simulink model "PMSMSim"  (R2024b)
settings: Solver=FixedStepAuto  StartTime=0  StopTime=15000  RelTol=1e-3
model workspace (MAT data in the model file):
  time = -1
libraries: deeplib x1
settings Model: SimulationMode=accelerator  Creator=skeshavm  LastModifiedBy=msatra
settings SolverCC: AlgebraicLoopSolver=TrustRegion
settings DataIOCC: SaveFormat=StructureWithTime  SaveOutput=off  SignalLogging=off  DSMLogging=off  SaveTime=off
settings OptimizationCC: DefaultParameterBehavior=Inlined  UseDivisionForNetSlopeComputation=on  GainParamInheritBuiltInType=on  UseFloatMulNetSlope=on  InlineInvariantSignals=on  StrengthReduction=on  PassReuseOutputArgsThreshold=0  ZeroExternalMemoryAtStartup=off  ZeroInternalMemoryAtStartup=off  InitFltsAndDblsToZero=on  EfficientFloat2IntCast=on  OptimizeBlockOrder=speed  OptimizationPriority=Speed  OptimizationCustomize=off  MultiThreadedLoops=on  AutoScheduleForLoops=on  DenormalBehavior=FlushToZero
settings DebuggingCC: InheritedTsInSrcMsg=none  MultiTaskCondExecSysMsg=none  MultiTaskRateTransMsg=warning  ParameterTunabilityLossMsg=error  UnconnectedInputMsg=warning  UnconnectedOutputMsg=warning  UnconnectedLineMsg=warning
settings HardwareCC: ProdLongLongMode=on  TargetLongLongMode=on
settings ModelReferenceCC: EnableRefExpFcnMdlSchedulingChecks=on
settings SFSimCC: MATLABDynamicMemAlloc=off  SimTargetLang=C++  GPUAcceleration=on  SimDLTargetLibrary=cudnn
settings RTWCC: Toolchain=Microsoft Visual C++ 2019 v16.0 | nmake (64-bit Windows)  BuildConfiguration=Faster Runs  TargetLang=C++  CheckMdlBeforeBuild=Warning  GPUErrorChecks=on  GPUComputeCapability=7.5  DLArmComputeVersion=19.05
settings CodeAppCC: ForceParamTrailComments=on  OperatorAnnotations=on
settings GRTTargetCC: TargetLangStandard=C++11 (ISO)  CodeInterfacePackaging=C++ class

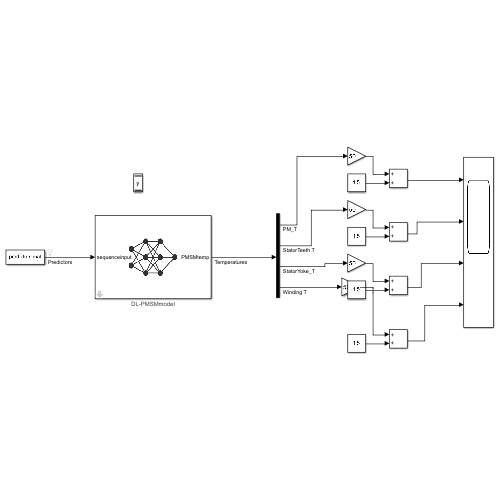
[thumbnail: Simulink's stored preview of the top-level diagram]
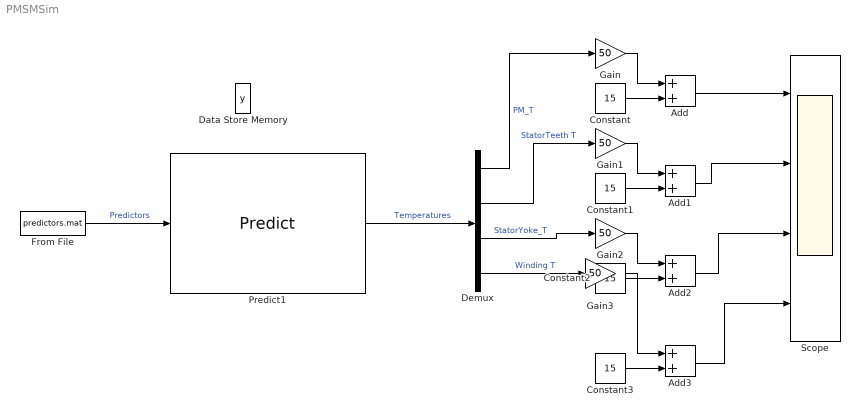
== system PMSMSim ==
  Add{,1..3} (4 alike) : Sum
  Constant{,1..3} (4 alike) : Constant  Value=15
  Data Store Memory : DataStoreMemory  DataStoreName=y  ReadBeforeWriteMsg=warning  WriteAfterWriteMsg=warning  WriteAfterReadMsg=warning  ShowAdditionalParam=off
  Demux : Demux
  From File : FromFile  FileName=predictors.mat  OutDataTypeStr=double
  Gain{,1..3} (4 alike) : Gain  Gain=50
  Predict1 : deeplib/Predict  Description=PMSM Predictor that uses DAG network  Network=Network from MAT-file  NetworkFunction=squeezenet  NetworkFilePath=C:\Mahaveer\Examples\AI with MBD_ROM_ Hands on Workshop\ROM of a PMSM Motor\Models\pmsmnet.mat  MiniBatchSize=1  InputDataFormats={ '', '' }  Predictions=on  Activations={}  ForceInterpretedSim=off  EnableDLNetwork=off  LastKnownNetworkFilePath=''  LastKnownNetworkTimeStamp=''
      settings: AttributesFormatString=DL-PMSMmodel
  Scope : Scope  NumInputPorts=4
  wires:
  Constant3/1 -> Add3/2
  Gain1/1 -> Add1/1
  Gain3/1 -> Add3/1
  Constant2/1 -> Add2/2
  Gain2/1 -> Add2/1
  Constant1/1 -> Add1/2
  Demux/2 -> Gain1/1  "StatorTeeth T"
  Demux/3 -> Gain2/1  "StatorYoke_T"
  From File/1 -> Predict1/1  "Predictors"
  Gain/1 -> Add/1
  Demux/4 -> Gain3/1  "Winding T"
  Add/1 -> Scope/1
  Add3/1 -> Scope/4
  Add1/1 -> Scope/2
  Demux/1 -> Gain/1  "PM_T"
  Constant/1 -> Add/2
  Add2/1 -> Scope/3
  Predict1/1 -> Demux/1  "Temperatures"
